simulink model "OvenController"  (R2013b)
settings: Solver=ode4  StartTime=0.0  StopTime=400  FixedStep=0.1  RelTol=1e-3
InitFcn:
  | %% useful unit conversions
  | CtoK = 273.15;		% converts a temperature in celsius to kelvin
  | 
  | %% air data from http://www.engineeringtoolbox.com/air-properties-d_156.html
  | air_data = [
  | -150	2.793	1.026	0.0116	3.08	8.21	0.76
  | -100	1.980	1.009	0.0160	5.95	5.82	0.74
  | -50	1.534	1.005	0.0204	9.55	4.51	0.725
  | 0	1.293	1.005	0.0243	13.30	3.67	0.715
  | 20	1.205	1.005	0.0257	15.11	3.43	0.713
  | 40	1.127	1.005	0.0271	16.97	3.20	0.711
  | 60	1.067	1.009	0.0285	18.90	3.00	0.709
  | 80	1.000	1.009	0.0299	20.94	2.83	0.708
  | 100	0.946	1.009	0.0314	23.06	2.68	0.703
  | 120	0.898	1.013	0.0328	25.23	2.55	0.70
  | 140	0.854	1.013	0.0343	27.55	2.43	0.695
  | 160	0.815	1.017	0.0358	29.85	2.32	0.69
  | 180	0.779	1.022	0.0372	32.29	2.21	0.69
  | 200	0.746	1.026	0.0386	34.63	2.11	0.685
  | 250	0.675	1.034	0.0421	41.17	1.91	0.68
  | 300	0.616	1.047	0.0454	47.85	1.75	0.68
  | 350	0.566	1.055	0.0485	55.05	1.61	0.68
  | 400	0.524	1.068	0.0515	62.53	1.49	0.68
  | ];
  | 
  | air_data_TEMP = 1;	% temperature (C)
  | air_data_RHO  = 2;	% density (kg/m^3)
  | air_data_CP   = 3;	% specific heat capacity (kJ/kgK)
  | 
  | %% the desired profile at the probe
  | temp_profile = [
  | 	0	20
  | 	60	200
  | 	100	100
  | 	300	100
  | 	360	20
  | 	];
  | temp_profile_TIME = 1;	% the time (s)
  | temp_profile_TEMP = 2;	% the desired probe temperature (C)
  | 
  | %% oven properties
  | oven_init_temp = 20;	% the initial temperature of the oven (C)
  | oven_volume = 0.5;		% volume of the oven (m^3)
  | burner_power = 4;		% heat output of the burner (kW)
  | oven_insulation = 0.01;	% conduction of the oven to the surrounding air (kW/K)
  | ambient_temp = 20;		% the ambient temperature (C)
  | ctl_tolerance = 1;		% the allowed delta temperature before the burner comes on (C)
  | 
  | target_init_temp = 20;	% the initial temperature of the target (C)
  | target_mass = 1;		% the mass of the target (kg)
  | target_c = 1;			% the specific heat of the target (kJ/kgK)
  | target_I = 1;			% the conductance between the oven air and the target (kW/K)
settings Model: Creator=etwigg  LastModifiedBy=etwigg
settings OptimizationCC: ExpressionDepthLimit=2147483647
settings DebuggingCC: StateNameClashWarn=warning

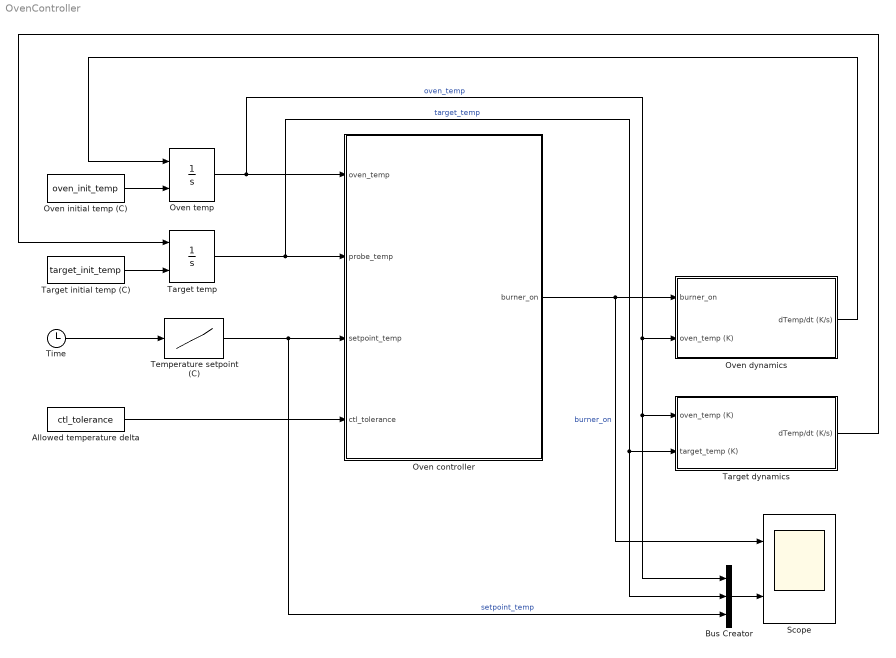
== system OvenController ==
  Allowed temperature delta : Constant  Value=ctl_tolerance
  Bus Creator : BusCreator  Inputs=3
  Oven controller : Stateflow chart  TreatAsAtomicUnit=on
  Oven dynamics : Subsystem
  Oven initial temp (C) : Constant  Value=oven_init_temp
  Oven temp : Integrator  InitialConditionSource=external
  Scope : Scope  NumInputPorts=2
      settings: YMin=-5~-5  YMax=5~5
  Target dynamics : Subsystem
  Target initial temp (C) : Constant  Value=target_init_temp
  Target temp : Integrator  InitialConditionSource=external
  Temperature setpoint (C) : Lookup_n-D  NumberOfTableDimensions=1  BreakpointsForDimension1=temp_profile(:,temp_profile_TIME)  Table=temp_profile(:,temp_profile_TEMP)  ExtrapMethod=Clip  UseLastTableValue=on  RndMeth=Simplest  InputSameDT=on
  Time : Clock
  wires:
  Time/1 -> Temperature setpoint (C)/1
  Temperature setpoint (C)/1 -> Bus Creator/3, Oven controller/3(setpoint_temp)  "setpoint_temp"
  Allowed temperature delta/1 -> Oven controller/4(ctl_tolerance)
  Oven temp/1 -> Bus Creator/1, Target dynamics/1(oven_temp (K)), Oven dynamics/2(oven_temp (K)), Oven controller/1(oven_temp)  "oven_temp"
  Oven controller/1(burner_on) -> Scope/1, Oven dynamics/1(burner_on)  "burner_on"
  Oven initial temp (C)/1 -> Oven temp/2
  Oven dynamics/1(dTemp/dt (K/s)) -> Oven temp/1
  Target dynamics/1(dTemp/dt (K/s)) -> Target temp/1
  Target temp/1 -> Bus Creator/2, Target dynamics/2(target_temp (K)), Oven controller/2(probe_temp)  "target_temp"
  Target initial temp (C)/1 -> Target temp/2
  Bus Creator/1 -> Scope/2

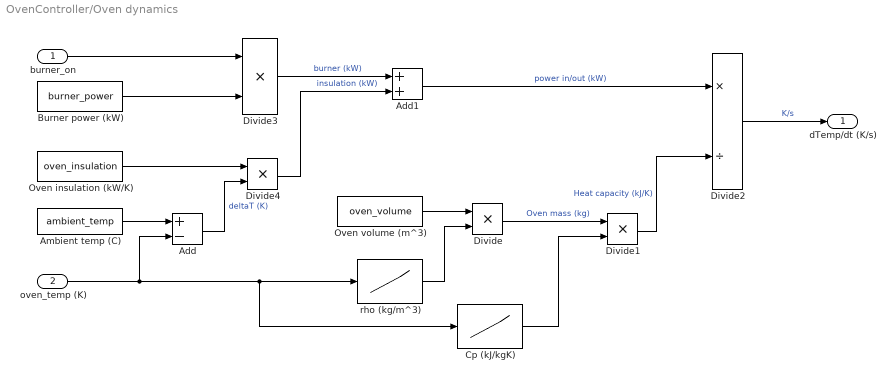
== system OvenController/Oven dynamics ==
  burner_on : Inport
  oven_temp (K) : Inport  Port=2
  Add : Sum  Inputs=+-
  Add1 : Sum
  Ambient temp (C) : Constant  Value=ambient_temp
  Burner power (kW) : Constant  Value=burner_power
  Cp (kJ/kgK) : Lookup_n-D  NumberOfTableDimensions=1  BreakpointsForDimension1=air_data(:,air_data_TEMP)  Table=air_data(:,air_data_CP)  DiagnosticForOutOfRangeInput=Warning  RndMeth=Simplest  InputSameDT=on
  Divide{,1,3..4} (4 alike) : Product  Inputs=**
  Divide2 : Product  Inputs=*/
  Oven insulation (kW/K) : Constant  Value=oven_insulation
  Oven volume (m^3) : Constant  Value=oven_volume
  rho (kg/m^3) : Lookup_n-D  NumberOfTableDimensions=1  BreakpointsForDimension1=air_data(:,air_data_TEMP)  Table=air_data(:,air_data_RHO)  DiagnosticForOutOfRangeInput=Warning  RndMeth=Simplest  InputSameDT=on
  dTemp/dt (K/s) : Outport
  wires:
  Add/1 -> Divide4/2  "deltaT (K)"
  Ambient temp (C)/1 -> Add/1
  burner_on/1 -> Divide3/1
  Oven insulation (kW/K)/1 -> Divide4/1
  Divide3/1 -> Add1/1  "burner (kW)"
  Oven volume (m^3)/1 -> Divide/1
  rho (kg/m^3)/1 -> Divide/2
  Divide1/1 -> Divide2/2  "Heat capacity (kJ/K)"
  Divide/1 -> Divide1/1  "Oven mass (kg)"
  Burner power (kW)/1 -> Divide3/2
  oven_temp (K)/1 -> Cp (kJ/kgK)/1, rho (kg/m^3)/1, Add/2
  Add1/1 -> Divide2/1  "power in/out (kW)"
  Divide4/1 -> Add1/2  "insulation (kW)"
  Cp (kJ/kgK)/1 -> Divide1/2
  Divide2/1 -> dTemp/dt (K/s)/1  "K/s"

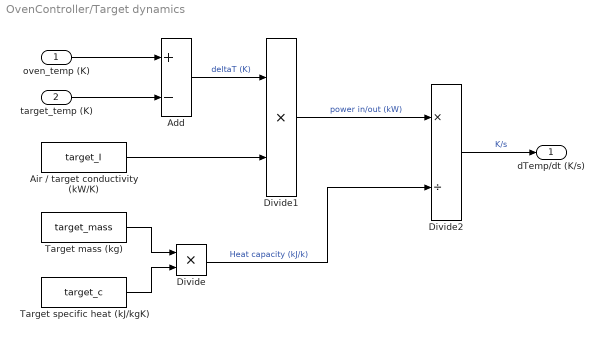
== system OvenController/Target dynamics ==
  oven_temp (K) : Inport
  target_temp (K) : Inport  Port=2
  Add : Sum  Inputs=+-
  Air / target conductivity (kW/K) : Constant  Value=target_I
  Divide : Product  Inputs=**
  Divide1 : Product  Inputs=**
  Divide2 : Product  Inputs=*/
  Target mass (kg) : Constant  Value=target_mass
  Target specific heat (kJ/kgK) : Constant  Value=target_c
  dTemp/dt (K/s) : Outport
  wires:
  oven_temp (K)/1 -> Add/1
  Target mass (kg)/1 -> Divide/1
  Divide/1 -> Divide2/2  "Heat capacity (kJ/k)"
  target_temp (K)/1 -> Add/2
  Divide1/1 -> Divide2/1  "power in/out (kW)"
  Divide2/1 -> dTemp/dt (K/s)/1  "K/s"
  Target specific heat (kJ/kgK)/1 -> Divide/2
  Add/1 -> Divide1/1  "deltaT (K)"
  Air / target conductivity (kW/K)/1 -> Divide1/2

== stateflow chart OvenController/Oven controller ==
  note: The burner state is toggled when the equilibrium temperature
      | exceeds the setpoint by ctl_tolerance.
  state BurnerOff
    entry: burner_on = 0;
  state BurnerOn
    entry: burner_on = 1;
  (default) -> BurnerOff
  BurnerOn -> BurnerOff : [calc_equilibrium() > setpoint_temp + ctl_tolerance]
  BurnerOff -> BurnerOn : [calc_equilibrium() < setpoint_temp - ctl_tolerance]
  data: equilibrium_temp function_output double; oven_temp input; probe_temp input; setpoint_temp input; burner_on output double; ctl_tolerance input
  function equilibrium_temp = calc_equilibrium:
    | function equilibrium_temp = calc_equilibrium
    | 
    | %% useful unit conversions
    | CtoK = 273.15;		% converts a temperature in celsius to kelvin
    | 
    | 
    | 
    | 
    | 
    | %% air data from http://www.engineeringtoolbox.com/air-properties-d_156.html
    | air_data = [
    | -150	2.793	1.026	0.0116	3.08	8.21	0.76
    | -100	1.980	1.009	0.0160	5.95	5.82	0.74
    | -50	1.534	1.005	0.0204	9.55	4.51	0.725
    | 0	1.293	1.005	0.0243	13.30	3.67	0.715
    | 20	1.205	1.005	0.0257	15.11	3.43	0.713
    | 40	1.127	1.005	0.0271	16.97	3.20	0.711
    | 60	1.067	1.009	0.0285	18.90	3.00	0.709
    | 80	1.000	1.009	0.0299	20.94	2.83	0.708
    | 100	0.946	1.009	0.0314	23.06	2.68	0.703
    | 120	0.898	1.013	0.0328	25.23	2.55	0.70
    | 140	0.854	1.013	0.0343	27.55	2.43	0.695
    | 160	0.815	1.017	0.0358	29.85	2.32	0.69
    | 180	0.779	1.022	0.0372	32.29	2.21	0.69
    | 200	0.746	1.026	0.0386	34.63	2.11	0.685
    | 250	0.675	1.034	0.0421	41.17	1.91	0.68
    | 300	0.616	1.047	0.0454	47.85	1.75	0.68
    | 350	0.566	1.055	0.0485	55.05	1.61	0.68
    | 400	0.524	1.068	0.0515	62.53	1.49	0.68
    | ];
    | 
    | air_data_TEMP = 1;	% temperature (C)
    | air_data_RHO  = 2;	% density (kg/m^3)
    | air_data_CP   = 3;	% specific heat capacity (kJ/kgK)
    | 
    | %% oven properties
    | oven_volume = 1.0;		% volume of the oven (m^3)
    | ambient_temp = 20;		% the ambient temperature (C)
    | 
    | target_mass = 1;		% the mass of the target (kg)
    | target_c = 1;			% the specific heat of the target (kJ/kgK)
    | 
    | %% calculate the energy in the oven and the target
    | oven_rho = interp1(air_data(:,air_data_TEMP), air_data(:,air_data_RHO), oven_temp);
    | oven_cp  = interp1(air_data(:,air_data_TEMP), air_data(:,air_data_CP), oven_temp);
    | 
    | oven_mass = oven_rho * oven_volume;
    | oven_capacity = oven_mass * oven_cp;
    | oven_U = oven_capacity * (oven_temp + CtoK);
    | 
    | target_capacity = target_mass * target_c;
    | target_U = target_capacity * (probe_temp + CtoK);
    | 
    | %% return the current equilibrium temperature
    | equilibrium_temp = ((oven_U + target_U) / (oven_capacity + target_capacity));
